simulink model "HvCoorn"  (R2022b)
settings: configuration reference "Icar05FusaMdlCfg" (kept outside this file)
undefined symbols (not defined in the file): BMSActSt_ACChrg, BMSActSt_DCChrg, BMSActSt_disconnect, BMSActSt_offline, BMSActSt_online, BMSActSt_undefined, BMSMainNegRlySt_Clsd_SC, BMSMainNegRlySt_Open_SC, BMSMainNegRlySt_StuckInClsd_SC, BMSMainNegRlySt_StuckInOpen_SC, BMSMainPosRlySt_Clsd_SC, BMSMainPosRlySt_Open_SC, BMSMainPosRlySt_StuckInClsd_SC, BMSPrecRlySt_StuckInOpen_SC, BMSReqSt_ACChrg, BMSReqSt_DCChrg, BMSReqSt_emergencyOffline, BMSReqSt_offline, BMSReqSt_online, Chrg_stCycleBookMod_SC, Chrg_stSingleBookMod_SC, CmpgMod_stInactv_SC, DCDCActSt_buck, DCDCActSt_connected, DCDCActSt_disconnected, DCDCReqSt_buck, DCDCReqSt_standby, EngStrtStop_RefuModDft_SC, EPBActSt_Appld_SC, GearLvr_stDrvGearD_SC, GearLvr_stDrvGearN_SC, GearLvr_stDrvGearP_SC, GearLvr_stDrvGearR_SC, hpp_bACChargeLinkIni_C, hpp_bACChargeLinkOKIni_C, hpp_bAcChgEnaIni_C, hpp_bAcChgPauseIni_C, hpp_bAcLinkTempErrIni_C, hpp_bBattWarmReqIni_C, hpp_bHvilHwErrIni_C, hpp_bHvilStOkIni_C, hpp_bHvRelayClsActIni_C, hpp_bHvRelayOpnActIni_C, hpp_bHvRelayStuckIni_C, hpp_bParked4ChDchgIni_C, hpp_bRemLvBatMntnReqIni_C, hpp_bStartUpReqIni_C, hpp_stHvilCanIni_C, hpp_stWarmTimeCfgRespIni_C, HvCoorn_bAuthEnaSwt_C, HvCoorn_bAuthFailSpdLimOvrd_C, HvCoorn_bAuthFailSpdLimOvrdVal_C, HvCoorn_bAuthStrt_C, HvCoorn_bBMSUnexpdDcnctFailEna_C, HvCoorn_bBuck2RdyBypDCDCEna_C, HvCoorn_bDCChrgFctCfg_C, HvCoorn_bDcChrgWkupEnaChrgLink_C, HvCoorn_bDCDcnct4ACEna_C, HvCoorn_bDCNotBuck2ShtdwnEna_C, HvCoorn_bDrvrLevNotRdyEna_C ... (+295)
libraries: ITKLib x213, simulink x61
(part 6 of 12)

== system HvCoorn/HvCoorn/HVP_HighVoltagePowerOnOffProcedure/A10_ShutDisCh2ShutECUCal ==
  note: Documentation
  HvCoorn_tiHVPStTimer : Inport
  HvCoorn_bHvRlyOpenAct : Inport  Port=2
  icfm_uAct : Inport  Port=3
  icdc_uHvAct : Inport  Port=4
  icfm_stMode : Inport  Port=5
  icrm_stMode : Inport  Port=6
  HvCoorn_bStartUpReq : Inport  Port=7
  HvCoorn_bHvOnFail : Inport  Port=8
  icobc_uHvDcAct : Inport  Port=9
  icfm_bUActSigErr : Inport  Port=10
  icobc_bUHvDcActSigErr : Inport  Port=11
  icdc_bUHvActSigErr : Inport  Port=12
  icbms_uHVBat : Inport  Port=13
  HvCoorn_bHvRlyStuck : Inport  Port=14
  icrm_uAct : Inport  Port=15
  icrm_bUActSigErr : Inport  Port=16
  VehCfg_bFrntMotByp : Inport  Port=17
  icfm_stActvDchrg : Inport  Port=18
  icrm_stActvDchrg : Inport  Port=19
  icisg_uAct : Inport  Port=20
  Add : Sum  Inputs=+-  SaturateOnIntegerOverflow=on
  Copyright : simulink/Model-Wide Utilities/Model Info  Frame=on  DisplayStringWithTags=|  HorizontalTextAlignment=Left  LeftAlignmentValue=0.02
      | © ITK Engineering Technology (Wu Xi) Co., Ltd. (ITKC)
      | 
      | Model Version: %<ModelVersion>
      | Date: %<LastModificationDate>
  FALSE : Constant  Description=FALSE  Value=0  OutDataTypeStr=boolean
      settings: AttributesFormatString=%<Description>
  InlineDescription : ITKLib/Special/InlineDescription  Tag=HideFromReport  Description=主动放电跳转至关ECU  ShowInLibBrowser=0  RefreshPar=0
      settings: SourceProductName=ITKC_Lib
  Logical Operator{1..2,5,11..12} (5 alike) : Logic  AllPortsSameDT=off  OutDataTypeStr=boolean
  Logical Operator3 : Logic  Operator=OR  Inputs=4  AllPortsSameDT=off  OutDataTypeStr=boolean
  Logical Operator4 : Logic  Inputs=3  AllPortsSameDT=off  OutDataTypeStr=boolean
  Logical Operator6 : Logic  Operator=OR  Inputs=4  AllPortsSameDT=off  OutDataTypeStr=boolean
  Logical Operator7 : Logic  Operator=NOT  Inputs=1  AllPortsSameDT=off  OutDataTypeStr=boolean
  Logical Operator8 : Logic  Operator=OR  Inputs=4  AllPortsSameDT=off  OutDataTypeStr=boolean
  Logical Operator9 : Logic  Operator=NOT  Inputs=1  AllPortsSameDT=off  OutDataTypeStr=boolean
  MinMax : MinMax  Function=max  Inputs=5  SaturateOnIntegerOverflow=on
  OR : Logic  Operator=OR  OutDataTypeStr=boolean
  Relational Operator1 : RelationalOperator  OutDataTypeStr=boolean  InputSameDT=off
  Relational Operator{2..3,6,8..10} (6 alike) : RelationalOperator  Operator===  OutDataTypeStr=boolean  InputSameDT=off
  Relational Operator4 : RelationalOperator  OutDataTypeStr=boolean  InputSameDT=off
  Relational Operator5 : RelationalOperator  Operator=>  OutDataTypeStr=boolean  InputSameDT=off
  Relational Operator7 : RelationalOperator  Operator=<  OutDataTypeStr=boolean  InputSameDT=off
  Switch : Switch  Criteria=u2 ~= 0  SaturateOnIntegerOverflow=off  InputSameDT=off
      settings: AttributesFormatString=Criteria : %<Criteria>
  Switch1 : Switch  Criteria=u2 ~= 0  SaturateOnIntegerOverflow=off  InputSameDT=off
      settings: AttributesFormatString=Criteria : %<Criteria>
  Switch2 : Switch  Criteria=u2 ~= 0  SaturateOnIntegerOverflow=off  InputSameDT=off
      settings: AttributesFormatString=Criteria : %<Criteria>
  TRUE : Constant  Description=TRUE  OutDataTypeStr=boolean
      settings: AttributesFormatString=%<Description>
  TRUE1 : Constant  Description=TRUE  OutDataTypeStr=boolean
      settings: AttributesFormatString=%<Description>
  Unit detailed design : simulink/Model-Wide Utilities/DocBlock  Tag=HideFromReport  DocumentType=Text
      content=|
      | SMiVCU-3304 - 电压差大使能高压标志位
      | <电池电压>大于<前电机电压>、<DCDC电压>、<OBC电压>、<后电机电压>超过一定值（HvCoorn_uHvDiffOnThrd_C），则激活[电压差大使能高压标志位]
      |
      | SMiVCU-3303 - MCU主动放电完成标志位
      | <前电机主动放电状态反馈>均为0x1：finished，则激活[MCU主动放电完成标志位]。
      |
      | SMiVCU-3308 - 主动放电跳转至关断ECU标志位
      | [高压继电器断开标志位]为1，且以下任一条件满足，则激活[主动放电跳转至关断ECU标志位]：
      | 1.[MCU主动放电完成标志位]为1；
      | 2.<前电机电压>、<DCDC电压>、<OBC电压>、<后电机电压>均小于一定值（HvCoorn_uMax4Shutdown_C，初始值60V）；
      | 3.<状态持续时间>大于一定值（HvCoorn_tiWait4DchaCanLost_C，5s）；
      | 4.[电压差大使能高压标志位]为1，且[上高压失败标志位]为0，且[上高压需求标志位]为1。
      |
      | SMiVCU-3310 - MCU主动放电失败标志位
      | <前电机主动放电状态反馈>均为0x3：Failure（两驱时屏蔽前电机）则激活[MCU主动放电失败标志位]；
      |
      | SMiVCU-3305 - 主动放电跳转至下电Error标志位
      | 以下任一条件满足，则激活[主动放电跳转至下电Error标志位]：
      | 1.<状态持续时间>大于等于一定值（HvCoorn_tiWait4HvDcha_C，初始值120s）；
      | 2.[高压继电器粘连标志位]为1；
      | 3.[MCU主动放电失败标志位]为1；
  icm_failure : Constant  Description=[8]  Value=MCUActSt_failure  OutDataTypeStr=uint8
      settings: AttributesFormatString=[8]
  icm_failure1 : Constant  Description=[8]  Value=MCUActSt_failure  OutDataTypeStr=uint8
      settings: AttributesFormatString=[8]
  icm_failure2 : Constant  Description=[3]  Value=MCUActvDcgrgSt_Failr_SC  OutDataTypeStr=uint8
      settings: AttributesFormatString=%<Description>
  icm_failure3 : Constant  Description=[3]  Value=MCUActvDcgrgSt_Failr_SC  OutDataTypeStr=uint8
      settings: AttributesFormatString=%<Description>
  icm_failure4 : Constant  Description=[1]  Value=MCUActvDcgrgSt_Cmpl_SC  OutDataTypeStr=uint8
      settings: AttributesFormatString=%<Description>
  icm_failure5 : Constant  Description=[1]  Value=MCUActvDcgrgSt_Cmpl_SC  OutDataTypeStr=uint8
      settings: AttributesFormatString=%<Description>
  sup_bEnaDCUStMan_C : Constant  Description=[0]  Value=HvCoorn_bEnaMCUStMan_C  OutDataTypeStr=boolean
      settings: AttributesFormatString=%<Description>
  sup_tiWait4DchaCanLost_C : Constant  Description=[5]  Value=HvCoorn_tiWait4DchaCanLost_C
      settings: AttributesFormatString=%<Description>
  sup_tiWait4HvDcha_C : Constant  Description=[120]  Value=HvCoorn_tiWait4HvDcha_C
      settings: AttributesFormatString=%<Description>
  sup_uHvDiffOnThres_C : Constant  Description=[70]  Value=HvCoorn_uHvDiffOnThrd_C
      settings: AttributesFormatString=%<Description>
  sup_uIpuShutdown_C : Constant  Description=[60]  Value=HvCoorn_uMax4Shutdown_C
      settings: AttributesFormatString=%<Description>
  HvCoorn_bShutDisCh2ShutECU : Outport  VectorParamsAs1DForOutWhenUnconnected=off
  HvCoorn_bShutDisCh2ShutErr : Outport  Port=2  VectorParamsAs1DForOutWhenUnconnected=off
  bVolDiffEnaHv : Outport  Port=3  VectorParamsAs1DForOutWhenUnconnected=off
  HvCoorn_bMCUActvDchrgCmpl : Outport  Port=4  VectorParamsAs1DForOutWhenUnconnected=off
  HvCoorn_bMCUActvDchrgErr : Outport  Port=5  VectorParamsAs1DForOutWhenUnconnected=off
  wires:
  Logical Operator3/1 -> HvCoorn_bShutDisCh2ShutErr/1  "HvCoorn_bShutDisCh2ShutErr"
  HvCoorn_tiHVPStTimer/1 -> [HvCoorn_tiHVPTimer], Relational Operator4/1
  sup_tiWait4HvDcha_C/1 -> Relational Operator4/2
  HvCoorn_bHvRlyOpenAct/1 -> Logical Operator2/1
  Logical Operator2/1 -> HvCoorn_bShutDisCh2ShutECU/1  "HvCoorn_bShutDisCh2ShutECU"
  sup_uIpuShutdown_C/1 -> Relational Operator7/2
  Relational Operator4/1 -> Logical Operator3/1
  HvCoorn_bHvRlyStuck/1 -> Logical Operator3/2
  icfm_stMode/1 -> Relational Operator2/1
  icm_failure/1 -> Relational Operator2/2
  Logical Operator1/1 -> Logical Operator3/3
  HvCoorn_bStartUpReq/1 -> Logical Operator4/3
  icfm_uAct/1 -> MinMax/1
  icdc_uHvAct/1 -> MinMax/2
  Relational Operator5/1 -> bVolDiffEnaHv/1, Logical Operator4/1
  Relational Operator7/1 -> Logical Operator5/1
  Logical Operator4/1 -> Logical Operator6/4
  Logical Operator6/1 -> Logical Operator2/2
  sup_bEnaDCUStMan_C/1 -> Logical Operator1/2
  HvCoorn_bHvOnFail/1 -> Logical Operator7/1
  Logical Operator7/1 -> Logical Operator4/2
  icobc_uHvDcAct/1 -> MinMax/3
  icbms_uHVBat/1 -> Add/1
  sup_uHvDiffOnThres_C/1 -> Relational Operator5/2
  Add/1 -> Relational Operator5/1
  MinMax/1 -> [HvCoorn_uMaxMCUDCOBC], Relational Operator7/1
  Logical Operator8/1 -> Logical Operator9/1
  icfm_bUActSigErr/1 -> Logical Operator8/1
  icobc_bUHvDcActSigErr/1 -> Logical Operator8/3
  icdc_bUHvActSigErr/1 -> Logical Operator8/2
  Logical Operator9/1 -> Logical Operator5/2
  Relational Operator1/1 -> Logical Operator6/3
  sup_tiWait4DchaCanLost_C/1 -> Relational Operator1/2
  Relational Operator2/1 -> Switch/3
  [HvCoorn_tiHVPTimer] -> Relational Operator1/1
  [HvCoorn_uMaxMCUDCOBC] -> Add/2
  icrm_uAct/1 -> MinMax/4
  icrm_bUActSigErr/1 -> Logical Operator8/4
  icm_failure1/1 -> Relational Operator3/2
  icrm_stMode/1 -> Relational Operator3/1
  Relational Operator3/1 -> OR/2
  OR/1 -> Logical Operator1/1
  Switch/1 -> OR/1
  VehCfg_bFrntMotByp/1 -> [VehCfg_bFrntMotByp], Switch/2
  FALSE/1 -> Switch/1
  TRUE1/1 -> Switch1/1
  icfm_stActvDchrg/1 -> [icfm_stActvDchrg], Relational Operator6/1
  Relational Operator6/1 -> Switch1/3
  icm_failure2/1 -> Relational Operator6/2
  Switch1/1 -> Logical Operator11/1
  icm_failure3/1 -> Relational Operator8/2
  icrm_stActvDchrg/1 -> [icrm_stActvDchrg], Relational Operator8/1
  Relational Operator8/1 -> Logical Operator11/2
  [VehCfg_bFrntMotByp] -> Switch1/2
  [VehCfg_bFrntMotByp] -> Switch2/2
  Relational Operator9/1 -> Switch2/3
  icm_failure4/1 -> Relational Operator9/2
  TRUE/1 -> Switch2/1
  [icfm_stActvDchrg] -> Relational Operator9/1
  Switch2/1 -> Logical Operator12/1
  icm_failure5/1 -> Relational Operator10/2
  [icrm_stActvDchrg] -> Relational Operator10/1
  Relational Operator10/1 -> Logical Operator12/2
  Logical Operator12/1 -> HvCoorn_bMCUActvDchrgCmpl/1, Logical Operator6/1
  Logical Operator11/1 -> Logical Operator3/4, HvCoorn_bMCUActvDchrgErr/1
  Logical Operator5/1 -> Logical Operator6/2
  icisg_uAct/1 -> MinMax/5

== system HvCoorn/HvCoorn/HVP_HighVoltagePowerOnOffProcedure/A11_ShutECU2AftRunCal ==
  note: Documentation
  HvCoorn_tiHVPStTimer : Inport
  icfm_uAct : Inport  Port=2
  HvCoorn_bStartUpReq : Inport  Port=3
  icdc_uHvAct : Inport  Port=4
  icrm_uAct : Inport  Port=5
  Copyright : simulink/Model-Wide Utilities/Model Info  Frame=on  DisplayStringWithTags=|  HorizontalTextAlignment=Left  LeftAlignmentValue=0.02
      | © ITK Engineering Technology (Wu Xi) Co., Ltd. (ITKC)
      | 
      | Model Version: %<ModelVersion>
      | Date: %<LastModificationDate>
  InlineDescription : ITKLib/Special/InlineDescription  Tag=HideFromReport  Description=关断ECU跳转至后运行  ShowInLibBrowser=0  RefreshPar=0
      settings: SourceProductName=ITKC_Lib
  Logical Operator1 : Logic  Inputs=3  AllPortsSameDT=off  OutDataTypeStr=boolean
  Logical Operator2 : Logic  Operator=OR  AllPortsSameDT=off  OutDataTypeStr=boolean
  Logical Operator3 : Logic  Operator=NOT  Inputs=1  AllPortsSameDT=off  OutDataTypeStr=boolean
  Max : MinMax  Function=max  Inputs=2  InputSameDT=on  SaturateOnIntegerOverflow=on
  Relational Operator1 : RelationalOperator  Operator=<  OutDataTypeStr=boolean  InputSameDT=off
  Relational Operator4 : RelationalOperator  OutDataTypeStr=boolean  InputSameDT=off
  Relational Operator7 : RelationalOperator  Operator=<  OutDataTypeStr=boolean  InputSameDT=off
  Unit detailed design : simulink/Model-Wide Utilities/DocBlock  Tag=HideFromReport  DocumentType=Text
      content=|
      | SMiVCU-3306 - 关断ECU跳转至后运行标志位
      | <状态持续时间>大于一定值（HvCoorn_tiShutDownDlyLih_C，初始值20s），或[上高压需求标志位]为0且<前后电机电压>、<DCDC电压>均小于一定值（HvCoorn_uMax4Shutdown_C，初始值60V），则激活[关断ECU跳转至后运行标志位]。
  sup_tiShutDownDlyLih_C : Constant  Description=[20]  Value=HvCoorn_tiShutDownDlyLih_C
      settings: AttributesFormatString=%<Description>
  sup_uIpuShutdown_C : Constant  Description=[60]  Value=HvCoorn_uMax4Shutdown_C
      settings: AttributesFormatString=%<Description>
  HvCoorn_bShutECU2AftRun : Outport  VectorParamsAs1DForOutWhenUnconnected=off
  wires:
  Logical Operator2/1 -> HvCoorn_bShutECU2AftRun/1  "HvCoorn_bShutECU2AftRun"
  icfm_uAct/1 -> Max/1
  sup_uIpuShutdown_C/1 -> Relational Operator7/2, Relational Operator1/2
  sup_tiShutDownDlyLih_C/1 -> Relational Operator4/2
  HvCoorn_tiHVPStTimer/1 -> Relational Operator4/1
  Relational Operator7/1 -> Logical Operator1/2
  Relational Operator4/1 -> Logical Operator2/2
  HvCoorn_bStartUpReq/1 -> Logical Operator3/1
  Logical Operator3/1 -> Logical Operator1/1
  Logical Operator1/1 -> Logical Operator2/1
  icdc_uHvAct/1 -> Relational Operator1/1
  Relational Operator1/1 -> Logical Operator1/3
  icrm_uAct/1 -> Max/2
  Max/1 -> Relational Operator7/1

== system HvCoorn/HvCoorn/HVP_HighVoltagePowerOnOffProcedure/A12_ShutECU2CommCal ==
  note: Documentation
  bVolDiffEnaHv : Inport
  HvCoorn_bStartUpReq : Inport  Port=2
  HvCoorn_bHvOnFail : Inport  Port=3
  HvCoorn_bDischargeErrOld : Inport  Port=4
  HvCoorn_bHvInitFail : Inport  Port=5
  Copyright : simulink/Model-Wide Utilities/Model Info  Frame=on  DisplayStringWithTags=|  HorizontalTextAlignment=Left  LeftAlignmentValue=0.02
      | © ITK Engineering Technology (Wu Xi) Co., Ltd. (ITKC)
      | 
      | Model Version: %<ModelVersion>
      | Date: %<LastModificationDate>
  InlineDescription : ITKLib/Special/InlineDescription  Tag=HideFromReport  Description=关断ECU跳转至通讯准备  ShowInLibBrowser=0  RefreshPar=0
      settings: SourceProductName=ITKC_Lib
  Logical Operator1 : Logic  Inputs=5  AllPortsSameDT=off  OutDataTypeStr=boolean
  Logical Operator2 : Logic  Operator=NOT  Inputs=1  AllPortsSameDT=off  OutDataTypeStr=boolean
  Logical Operator3 : Logic  Operator=NOT  Inputs=1  AllPortsSameDT=off  OutDataTypeStr=boolean
  Logical Operator4 : Logic  Operator=NOT  Inputs=1  AllPortsSameDT=off  OutDataTypeStr=boolean
  Unit detailed design : simulink/Model-Wide Utilities/DocBlock  Tag=HideFromReport  DocumentType=Text
      content=|
      | SMiVCU-3309 - 关断ECU跳转至通讯准备标志位
      | 以下条件全部满足，则激活[关断ECU跳转至通讯准备标志位]：
      | 1.[上高压需求标志位]为1；
      | 2.[上高压失败标志位]为0；
      | 3.[MCU主动放电失败标志位]为0；
      | 4.[高压初始化失败标志位]为0；
      | 5.[电压差大使能高压标志位]为1；
  HvCoorn_bShutECU2Comm : Outport  VectorParamsAs1DForOutWhenUnconnected=off
  wires:
  HvCoorn_bHvOnFail/1 -> Logical Operator3/1
  HvCoorn_bDischargeErrOld/1 -> Logical Operator4/1
  HvCoorn_bStartUpReq/1 -> Logical Operator1/1
  Logical Operator3/1 -> Logical Operator1/2
  Logical Operator4/1 -> Logical Operator1/3
  Logical Operator1/1 -> HvCoorn_bShutECU2Comm/1  "HvCoorn_bShutECU2Comm"
  HvCoorn_bHvInitFail/1 -> Logical Operator2/1
  Logical Operator2/1 -> Logical Operator1/4
  bVolDiffEnaHv/1 -> Logical Operator1/5

== system HvCoorn/HvCoorn/HVP_HighVoltagePowerOnOffProcedure/A13_AftRun2NetManCal ==
  note: Documentation
  HvCoorn_tiHVPTimer : Inport
  HvCoorn_bStartUpReq : Inport  Port=2
  EngStrtStop_stRefuMod : Inport  Port=3
  Calibration1 : Constant  Description=[0]  Value=EngStrtStop_RefuModDft_SC  SampleTime=-1
      settings: AttributesFormatString=%<Description>
  Calibration2 : Constant  Description=[300]  Value=HvCoorn_tiRefuModOvti2NetManDly_C  SampleTime=-1
      settings: AttributesFormatString=%<Description>
  Copyright : simulink/Model-Wide Utilities/Model Info  Frame=on  DisplayStringWithTags=|  HorizontalTextAlignment=Left  LeftAlignmentValue=0.02
      | © ITK Engineering Technology (Wu Xi) Co., Ltd. (ITKC)
      | 
      | Model Version: %<ModelVersion>
      | Date: %<LastModificationDate>
  Equal1 : RelationalOperator  Operator===  OutDataTypeStr=boolean
  InlineDescription : ITKLib/Special/InlineDescription  Tag=HideFromReport  Description=后运行跳转至网络保持  ShowInLibBrowser=0  RefreshPar=0
      settings: SourceProductName=ITKC_Lib
  Logical Operator5 : Logic  Operator=NOT  Inputs=1  AllPortsSameDT=off  OutDataTypeStr=boolean
  Logical Operator6 : Logic  Inputs=3  AllPortsSameDT=off  OutDataTypeStr=boolean
  Not : Logic  Operator=NOT  AllPortsSameDT=off  OutDataTypeStr=boolean
  OR : Logic  Operator=OR  Inputs=3  OutDataTypeStr=boolean
  Relational Operator4 : RelationalOperator  Operator=>  OutDataTypeStr=boolean  InputSameDT=off
  TaskTime_s3 : Constant  Value=TaskTime_10ms
      settings: AttributesFormatString=[0.01]
  TurnOnDelayVari1 : ITKLib/TimeCounter/TurnOnDelayVari
      settings: AttributesFormatString=TurnOnDelay  SourceProductName=ITKC_Lib
  Unit detailed design : simulink/Model-Wide Utilities/DocBlock  Tag=HideFromReport  DocumentType=Text
      content=|
      | SMiVCU-3313 - 后运行跳转至网络保持标志位
      | <状态持续时间>大于一定值（HvCoorn_tiWaitChrgFullShutdown_C，1s）且[上高压需求标志位]为0，则激活[后运行跳转至网络保持标志位]。
  sup_tiWaitChgFullShutdown_C : Constant  Description=[1]  Value=HvCoorn_tiWaitChrgFullShutdown_C
      settings: AttributesFormatString=%<Description>
  sup_tiWaitChgFullShutdown_C1 : Constant  Description=[0]  Value=HvCoorn_bRefuModOvti2NetManShd_C
      settings: AttributesFormatString=%<Description>
  HvCoorn_bAftRun2NetMan : Outport  VectorParamsAs1DForOutWhenUnconnected=off
  wires:
  HvCoorn_tiHVPTimer/1 -> Relational Operator4/1
  sup_tiWaitChgFullShutdown_C/1 -> Relational Operator4/2
  Relational Operator4/1 -> Logical Operator6/1
  HvCoorn_bStartUpReq/1 -> Logical Operator5/1
  Logical Operator6/1 -> HvCoorn_bAftRun2NetMan/1  "HvCoorn_bAftRun2NetMan"
  Logical Operator5/1 -> Logical Operator6/2
  EngStrtStop_stRefuMod/1 -> Equal1/1
  Calibration1/1 -> Equal1/2
  Equal1/1 -> OR/2, Not/1
  Calibration2/1 -> TurnOnDelayVari1/3
  TaskTime_s3/1 -> TurnOnDelayVari1/2
  Not/1 -> TurnOnDelayVari1/1
  TurnOnDelayVari1/1 -> OR/3
  OR/1 -> Logical Operator6/3
  sup_tiWaitChgFullShutdown_C1/1 -> OR/1

== system HvCoorn/HvCoorn/HVP_HighVoltagePowerOnOffProcedure/A14_NetMan2PwrShutCal ==
  VCCM_bNetMaintn : Inport
  HvCoorn_tiHVPStTimer : Inport  Port=2
  HvCoorn_stHVPOld : Inport  Port=3
  AND : Logic  OutDataTypeStr=boolean
  Logical Operator4 : Logic  Operator=OR  Inputs=3  AllPortsSameDT=off  OutDataTypeStr=boolean
  Not : Logic  Operator=NOT  AllPortsSameDT=off  OutDataTypeStr=boolean
  Relational Operator15 : RelationalOperator  Operator===  OutDataTypeStr=boolean  InputSameDT=off
  Relational Operator4 : RelationalOperator  Operator=>  OutDataTypeStr=boolean  InputSameDT=off
  Wait4MindChange : Constant  Value=125  OutDataTypeStr=uint8
  sup_bLlswShutDownMan_C : Constant  Description=[0]  Value=HvCoorn_bLlswShutDownMan_C  OutDataTypeStr=boolean
      settings: AttributesFormatString=%<Description>
  sup_tiTimeOutStandbyRdyHv_C : Constant  Description=[120]  Value=HvCoorn_tiTimeOutNetMan_C
      settings: AttributesFormatString=%<Description>
  HvCoorn_bNetMan2PwrShut : Outport  VectorParamsAs1DForOutWhenUnconnected=off
  wires:
  VCCM_bNetMaintn/1 -> Not/1
  sup_bLlswShutDownMan_C/1 -> Logical Operator4/2
  Logical Operator4/1 -> HvCoorn_bNetMan2PwrShut/1  "HvCoorn_bNetMan2PwrShut"
  Not/1 -> Logical Operator4/1
  HvCoorn_tiHVPStTimer/1 -> Relational Operator4/1
  Relational Operator4/1 -> AND/1
  Relational Operator15/1 -> AND/2
  AND/1 -> Logical Operator4/3
  HvCoorn_stHVPOld/1 -> Relational Operator15/1
  sup_tiTimeOutStandbyRdyHv_C/1 -> Relational Operator4/2
  Wait4MindChange/1 -> Relational Operator15/2

== system HvCoorn/HvCoorn/HVP_HighVoltagePowerOnOffProcedure/A15_Wake2NetManCal ==
  note: Documentation
  HvCoorn_bStartUpReq : Inport
  HvCoorn_tiHVPTimer : Inport  Port=2
  Copyright : simulink/Model-Wide Utilities/Model Info  Frame=on  DisplayStringWithTags=|  HorizontalTextAlignment=Left  LeftAlignmentValue=0.02
      | © ITK Engineering Technology (Wu Xi) Co., Ltd. (ITKC)
      | 
      | Model Version: %<ModelVersion>
      | Date: %<LastModificationDate>
  InlineDescription : ITKLib/Special/InlineDescription  Tag=HideFromReport  Description=唤醒跳转至网络保持  ShowInLibBrowser=0  RefreshPar=0
      settings: SourceProductName=ITKC_Lib
  Logical Operator2 : Logic  AllPortsSameDT=off  OutDataTypeStr=boolean
  Logical Operator5 : Logic  Operator=NOT  Inputs=1  AllPortsSameDT=off  OutDataTypeStr=boolean
  Relational Operator4 : RelationalOperator  Operator=>  OutDataTypeStr=boolean  InputSameDT=off
  Unit detailed design : simulink/Model-Wide Utilities/DocBlock  Tag=HideFromReport  DocumentType=Text
      content=|
      | <状态持续时间>大于一定值（HvCoorn_tiKeyOnChk_C，0.05s）且[上高压需求标志位]为0，则激活[唤醒至网络保持标志位]。
  sup_tiKeyOnCheck_C : Constant  Description=[5]  Value=HvCoorn_tiKeyOnChk_C
      settings: AttributesFormatString=%<Description>
  HvCoorn_bWake2NetMan : Outport  VectorParamsAs1DForOutWhenUnconnected=off
  wires:
  HvCoorn_bStartUpReq/1 -> Logical Operator5/1
  Logical Operator2/1 -> HvCoorn_bWake2NetMan/1  "HvCoorn_bWake2NetMan"
  HvCoorn_tiHVPTimer/1 -> Relational Operator4/1
  sup_tiKeyOnCheck_C/1 -> Relational Operator4/2
  Logical Operator5/1 -> Logical Operator2/1
  Relational Operator4/1 -> Logical Operator2/2

== system HvCoorn/HvCoorn/HVP_HighVoltagePowerOnOffProcedure/A16_Init2AftRunCal ==
  note: Documentation
  HvCoorn_bStartUpReq : Inport
  HvCoorn_tiHVPTimer : Inport  Port=2
  Copyright : simulink/Model-Wide Utilities/Model Info  Frame=on  DisplayStringWithTags=|  HorizontalTextAlignment=Left  LeftAlignmentValue=0.02
      | © ITK Engineering Technology (Wu Xi) Co., Ltd. (ITKC)
      | 
      | Model Version: %<ModelVersion>
      | Date: %<LastModificationDate>
  InlineDescription : ITKLib/Special/InlineDescription  Tag=HideFromReport  Description=初始化跳转至后运行  ShowInLibBrowser=0  RefreshPar=0
      settings: SourceProductName=ITKC_Lib
  Logical Operator2 : Logic  AllPortsSameDT=off  OutDataTypeStr=boolean
  Logical Operator5 : Logic  Operator=NOT  Inputs=1  AllPortsSameDT=off  OutDataTypeStr=boolean
  Relational Operator4 : RelationalOperator  Operator=>  OutDataTypeStr=boolean  InputSameDT=off
  Unit detailed design : simulink/Model-Wide Utilities/DocBlock  Tag=HideFromReport  DocumentType=Text
      content=|
      | <状态持续时间>大于一定值（HvCoorn_tiWaitIgnOff_C，5s）且[上高压需求标志位]为0，则激活[初始化跳转至后运行标志位]。
  sup_tiWaitIgnOff_C : Constant  Description=[5]  Value=HvCoorn_tiWaitIgnOff_C
      settings: AttributesFormatString=%<Description>
  HvCoorn_bInit2AftRun : Outport  VectorParamsAs1DForOutWhenUnconnected=off
  wires:
  Relational Operator4/1 -> Logical Operator2/2
  Logical Operator5/1 -> Logical Operator2/1
  sup_tiWaitIgnOff_C/1 -> Relational Operator4/2
  HvCoorn_tiHVPTimer/1 -> Relational Operator4/1
  Logical Operator2/1 -> HvCoorn_bInit2AftRun/1  "HvCoorn_bInit2AftRun"
  HvCoorn_bStartUpReq/1 -> Logical Operator5/1

== system HvCoorn/HvCoorn/HVP_HighVoltagePowerOnOffProcedure/A17_EmergencyShutDownCal ==
  note: Documentation
  HvCoorn_tiHVPStTimer : Inport
  HvCoorn_bHvRlyStuck : Inport  Port=2
  HvCoorn_bHvRlyOpenAct : Inport  Port=3
  icfm_uAct : Inport  Port=4
  icdc_uHvAct : Inport  Port=5
  icfm_stMode : Inport  Port=6
  icbms_iHVBat : Inport  Port=7
  HvCoorn_bStartUpReq : Inport  Port=8
  icfm_nAct : Inport  Port=9
  HvCoorn_stHVPOld : Inport  Port=10
  ved_bHvShtdwn : Inport  Port=11
  icobc_uHvDcAct : Inport  Port=12
  icfm_bUActSigErr : Inport  Port=13
  icobc_bUHvDcActSigErr : Inport  Port=14
  icdc_bUHvActSigErr : Inport  Port=15
  icrm_nAct : Inport  Port=16
  icrm_bUActSigErr : Inport  Port=17
  icrm_uAct : Inport  Port=18
  icrm_stMode : Inport  Port=19
  HvCoorn_bMCUActvDchrgCmpl : Inport  Port=20
  HvCoorn_bMCUActvDchrgErr : Inport  Port=21
  Abs : Abs
  Abs1 : Abs
  Abs2 : Abs
  Copyright : simulink/Model-Wide Utilities/Model Info  Frame=on  DisplayStringWithTags=|  HorizontalTextAlignment=Left  LeftAlignmentValue=0.02
      | © ITK Engineering Technology (Wu Xi) Co., Ltd. (ITKC)
      | 
      | Model Version: %<ModelVersion>
      | Date: %<LastModificationDate>
  EmWait4KeyOff : Constant  Description=EmWait4KeyOff  Value=156  OutDataTypeStr=uint8
      settings: AttributesFormatString=|
      | %<OutDataTypeStr>
      | %<Description>
  InlineDescription : ITKLib/Special/InlineDescription  Tag=HideFromReport  Description=紧急下电  ShowInLibBrowser=0  RefreshPar=0
      settings: SourceProductName=ITKC_Lib
  Logical Operator1 : Logic  Operator=OR  Inputs=3  AllPortsSameDT=off  OutDataTypeStr=boolean
  Logical Operator{4,6,8,11} (4 alike) : Logic  AllPortsSameDT=off  OutDataTypeStr=boolean
  Logical Operator12 : Logic  Operator=OR  Inputs=4  AllPortsSameDT=off  OutDataTypeStr=boolean
  Logical Operator13 : Logic  Operator=NOT  Inputs=1  AllPortsSameDT=off  OutDataTypeStr=boolean
  Logical Operator2 : Logic  Operator=NOT  Inputs=1  AllPortsSameDT=off  OutDataTypeStr=boolean
  Logical Operator3 : Logic  Operator=OR  Inputs=4  AllPortsSameDT=off  OutDataTypeStr=boolean
  Logical Operator5 : Logic  Operator=OR  AllPortsSameDT=off  OutDataTypeStr=boolean
  Logical Operator7 : Logic  Operator=NOT  Inputs=1  AllPortsSameDT=off  OutDataTypeStr=boolean
  Logical Operator9 : Logic  Inputs=3  AllPortsSameDT=off  OutDataTypeStr=boolean
  Max : MinMax  Function=max  Inputs=2  InputSameDT=on  SaturateOnIntegerOverflow=on
  MinMax : MinMax  Function=max  Inputs=4  SaturateOnIntegerOverflow=on
  OR : Logic  Operator=OR  OutDataTypeStr=boolean
  OR1 : Logic  Operator=OR  OutDataTypeStr=boolean
  Relational Operator1 : RelationalOperator  OutDataTypeStr=boolean  InputSameDT=off
  Relational Operator10 : RelationalOperator  Operator=<=  OutDataTypeStr=boolean  InputSameDT=off
  Relational Operator11 : RelationalOperator  Operator=<  OutDataTypeStr=boolean  InputSameDT=off
  Relational Operator2 : RelationalOperator  OutDataTypeStr=boolean  InputSameDT=off
  Relational Operator3 : RelationalOperator  Operator===  OutDataTypeStr=boolean  InputSameDT=off
  Relational Operator4 : RelationalOperator  Operator=>  OutDataTypeStr=boolean  InputSameDT=off
  Relational Operator5 : RelationalOperator  OutDataTypeStr=boolean  InputSameDT=off
  Relational Operator6 : RelationalOperator  Operator=>  OutDataTypeStr=boolean  InputSameDT=off
  Relational Operator7 : RelationalOperator  Operator=>  OutDataTypeStr=boolean  InputSameDT=off
  Relational Operator8 : RelationalOperator  Operator=<  OutDataTypeStr=boolean  InputSameDT=off
  Relational Operator9 : RelationalOperator  Operator===  OutDataTypeStr=boolean  InputSameDT=off
  Unit detailed design : simulink/Model-Wide Utilities/DocBlock  Tag=HideFromReport  DocumentType=Text
      content=|
      | SMiVCU-3320 - 紧急下电初始化跳转至断高压标志位
      | <电池电流>的绝对值小于一定值（HvCoorn_iBatMax4RlyOpen_C，5s）或<状态持续时间>大于一定值（HvCoorn_tiHvOpenDlyEmerg_C，5s），则激活[紧急下电初始化跳转至断高压标志位]。
      |
      |
      | SMiVCU-3321 - 紧急下电放电跳转至放电Error标志位
      | 以下任一条件满足，则激活[紧急下电放电跳转至放电Error标志位]：
      | 1.<状态持续时间>大于一定值（HvCoorn_tiWait4HvDcha_C，120s）；
      | 2.[MCU主动放电失败标志位]为1；
      | 3.[高压继电器粘连标志位]为1；
      |
      | SMiVCU-3329 - 紧急下电等待KeyOff跳转至网络保持标志位
      | <状态持续时间>大于一定值（HvCoorn_tiWait4LlswEolShutdown_C，10s）且[上高压需求标志位]为0，则激活[紧急下电等待KeyOff跳转至网络保持标志位]。
      |
      | SMiVCU-3327 - 紧急下电放电跳转至等待KeyOff标志位
      | 以下条件全部满足，则激活[紧急下电放电跳转至等待KeyOff标志位]：
      | 1.[MCU主动放电完成标志位]为1；
      | 2.<前电机电压>、<DCDC电压>、<OBC电压>、<后电机电压>均小于一定值（HvCoorn_uThd4EmergShutdown_C，初始值60V）；
      | 3.<状态持续时间>大于一定值（HvCoorn_tiWait4DchaCanLost_C，5s）；
      |
      | SMiVCU-3331 - 紧急下电退出标志位
      | 满足以下全部条件，则激活[紧急下电退出标志位]:
      | 1.[紧急下电放电跳转至等待KeyOff标志位]为1；
      | 2.上一时刻<高压系统状态>大于156；
      | 3.[下电请求标志位]为0；
      |
      | SMiVCU-3333 - 紧急下电断高压跳转至主动放电标志位
      | [高压继电器断开标志位]为1，且<前后电机转速>的绝对值均小于一定值（HvCoorn_nMotThrd4DChrg_C，60rpm），则激活[紧急下电断高压跳转至主动放电标志位]
  icm_failure : Constant  Description=[8]  Value=MCUActSt_failure  OutDataTypeStr=uint8
      settings: AttributesFormatString=[8]
  icm_failure1 : Constant  Description=[8]  Value=MCUActSt_failure  OutDataTypeStr=uint8
      settings: AttributesFormatString=[8]
  sup_bEmEnaDCUStMan_C : Constant  Description=[0]  Value=HvCoorn_bEmEnaMCUStMan_C  OutDataTypeStr=boolean
      settings: AttributesFormatString=%<Description>
  sup_iBatMax4RlyOpn_C : Constant  Description=[5]  Value=HvCoorn_iBatMax4RlyOpen_C
      settings: AttributesFormatString=%<Description>
  sup_nMotThres4Dcha_C : Constant  Description=[30000]  Value=HvCoorn_nMotEmShutHv2DChrg_C
      settings: AttributesFormatString=%<Description>
  sup_tiHvesOpDlyEmerg_C : Constant  Description=[0.2]  Value=HvCoorn_tiHvOpenDlyEmerg_C
      settings: AttributesFormatString=%<Description>
  sup_tiWait4DchaCanLost_C : Constant  Description=[5]  Value=HvCoorn_tiWait4DchaCanLost_C
      settings: AttributesFormatString=%<Description>
  sup_tiWait4HvDcha_C : Constant  Description=[120]  Value=HvCoorn_tiWait4HvDcha_C
      settings: AttributesFormatString=%<Description>
  sup_tiWait4LlswEolShutdown_C : Constant  Description=[10]  Value=HvCoorn_tiWait4LlswEolShutdown_C
      settings: AttributesFormatString=%<Description>
  sup_tiWait4LlswEolShutdown_C1 : Constant  Description=[0.2]  Value=HvCoorn_tiWait4EmShutHv2DChrg_C
      settings: AttributesFormatString=%<Description>
  sup_uThresEmerg_C : Constant  Description=[60]  Value=HvCoorn_uThd4EmergShutdown_C
      settings: AttributesFormatString=%<Description>
  HvCoorn_bEmIni2ShutHV : Outport  VectorParamsAs1DForOutWhenUnconnected=off
  HvCoorn_bEmShutHv2DisCh : Outport  Port=2  VectorParamsAs1DForOutWhenUnconnected=off
  HvCoorn_bEmDisCh2WaitKeyOff : Outport  Port=3  VectorParamsAs1DForOutWhenUnconnected=off
  HvCoorn_bEmDisCh2Err : Outport  Port=4  VectorParamsAs1DForOutWhenUnconnected=off
  HvCoorn_bEmWaitKeyOff2NetMan : Outport  Port=5  VectorParamsAs1DForOutWhenUnconnected=off
  HvCoorn_bEmShutHeal : Outport  Port=6  VectorParamsAs1DForOutWhenUnconnected=off
  wires:
  sup_tiHvesOpDlyEmerg_C/1 -> Relational Operator4/2
  Logical Operator5/1 -> HvCoorn_bEmIni2ShutHV/1
  sup_tiWait4HvDcha_C/1 -> Relational Operator2/2
  Logical Operator3/1 -> HvCoorn_bEmDisCh2Err/1
  sup_tiWait4LlswEolShutdown_C/1 -> Relational Operator7/2
  Logical Operator1/1 -> HvCoorn_bEmDisCh2WaitKeyOff/1, Logical Operator9/1
  Relational Operator2/1 -> Logical Operator3/1
  HvCoorn_bHvRlyStuck/1 -> Logical Operator3/3
  icfm_stMode/1 -> Relational Operator9/1
  icm_failure/1 -> Relational Operator9/2
  Logical Operator6/1 -> Logical Operator3/4
  sup_nMotThres4Dcha_C/1 -> Relational Operator10/2
  Abs/1 -> Max/1
  icfm_nAct/1 -> Abs/1
  Relational Operator10/1 -> Logical Operator4/2
  HvCoorn_bHvRlyOpenAct/1 -> Logical Operator4/1
  sup_iBatMax4RlyOpn_C/1 -> Relational Operator11/2
  Abs1/1 -> Relational Operator11/1
  icbms_iHVBat/1 -> Abs1/1
  Relational Operator11/1 -> Logical Operator5/1
  Relational Operator4/1 -> Logical Operator5/2
  sup_bEmEnaDCUStMan_C/1 -> Logical Operator6/2
  Relational Operator9/1 -> OR/1
  HvCoorn_bStartUpReq/1 -> Logical Operator7/1
  Relational Operator7/1 -> Logical Operator8/1
  Logical Operator8/1 -> HvCoorn_bEmWaitKeyOff2NetMan/1
  Logical Operator7/1 -> Logical Operator8/2
  EmWait4KeyOff/1 -> Relational Operator1/2
  HvCoorn_stHVPOld/1 -> Relational Operator1/1
  ved_bHvShtdwn/1 -> Logical Operator2/1
  Relational Operator1/1 -> Logical Operator9/2
  Logical Operator2/1 -> Logical Operator9/3
  Logical Operator9/1 -> HvCoorn_bEmShutHeal/1
  sup_uThresEmerg_C/1 -> Relational Operator8/2
  icfm_uAct/1 -> MinMax/1
  icdc_uHvAct/1 -> MinMax/2
  Relational Operator8/1 -> Logical Operator11/1
  icobc_uHvDcAct/1 -> MinMax/3
  MinMax/1 -> Relational Operator8/1
  Logical Operator12/1 -> Logical Operator13/1
  icfm_bUActSigErr/1 -> Logical Operator12/1
  icobc_bUHvDcActSigErr/1 -> Logical Operator12/3
  icdc_bUHvActSigErr/1 -> Logical Operator12/2
  Logical Operator13/1 -> Logical Operator11/2
  sup_tiWait4DchaCanLost_C/1 -> Relational Operator5/2
  HvCoorn_tiHVPStTimer/1 -> [HvCoorn_tiHVPTimer], Relational Operator2/1, Relational Operator4/1
  [HvCoorn_tiHVPTimer] -> Relational Operator7/1
  [HvCoorn_tiHVPTimer] -> Relational Operator5/1
  icrm_nAct/1 -> Abs2/1
  Abs2/1 -> Max/2
  Max/1 -> Relational Operator10/1
  icrm_bUActSigErr/1 -> Logical Operator12/4
  icrm_uAct/1 -> MinMax/4
  icm_failure1/1 -> Relational Operator3/2
  icrm_stMode/1 -> Relational Operator3/1
  Relational Operator3/1 -> OR/2
  OR/1 -> Logical Operator6/1
  HvCoorn_bMCUActvDchrgErr/1 -> Logical Operator3/2
  HvCoorn_bMCUActvDchrgCmpl/1 -> Logical Operator1/1
  Logical Operator11/1 -> Logical Operator1/2
  Relational Operator5/1 -> Logical Operator1/3
  [HvCoorn_tiHVPTimer] -> Relational Operator6/1
  sup_tiWait4LlswEolShutdown_C1/1 -> Relational Operator6/2
  Logical Operator4/1 -> OR1/1
  Relational Operator6/1 -> OR1/2
  OR1/1 -> HvCoorn_bEmShutHv2DisCh/1

== system HvCoorn/HvCoorn/HVP_HighVoltagePowerOnOffProcedure/A18_ShutDownReqCal ==
  note: This subsystem calculates vehicle high voltage shut down flag and emergency shut down flag, based on vehicle eror level signal.
  note: Documentation
  ved_bEmgcyHvShtdwn : Inport
  HvCoorn_stHVPOld : Inport  Port=2
  Copyright : simulink/Model-Wide Utilities/Model Info  Frame=on  DisplayStringWithTags=|  HorizontalTextAlignment=Left  LeftAlignmentValue=0.02
      | © ITK Engineering Technology (Wu Xi) Co., Ltd. (ITKC)
      | 
      | Model Version: %<ModelVersion>
      | Date: %<LastModificationDate>
  InlineDescription : ITKLib/Special/InlineDescription  Tag=HideFromReport  Description=故障下高压  ShowInLibBrowser=0  RefreshPar=0
      settings: SourceProductName=ITKC_Lib
  Logical Operator1 : Logic  Inputs=3  AllPortsSameDT=off  OutDataTypeStr=boolean
  NormShut2 : Constant  Description=HvContactorRequest  Value=12  OutDataTypeStr=uint8
      settings: AttributesFormatString=|
      | %<OutDataTypeStr>
      | %<Description>
  NormShut3 : Constant  Description=Shutdown_HV  Value=101  OutDataTypeStr=uint8
      settings: AttributesFormatString=|
      | %<OutDataTypeStr>
      | %<Description>
  Relational Operator12 : RelationalOperator  OutDataTypeStr=boolean  InputSameDT=off
  Relational Operator3 : RelationalOperator  Operator=<=  OutDataTypeStr=boolean  InputSameDT=off
  Unit detailed design : simulink/Model-Wide Utilities/DocBlock  Tag=HideFromReport  DocumentType=Text
      content=|
      | SMiVCU-3772 - 故障下高压
      | 若<整车故障等级>大于等于4，则激活[下电请求标志位]。
      |
      | 若<整车故障等级>等于5，且上一时刻<高压系统状态>在12~101之间，则激活[紧急下电请求]
  HvCoorn_bEmgcyShutDownReq : Outport  VectorParamsAs1DForOutWhenUnconnected=off
  wires:
  Logical Operator1/1 -> HvCoorn_bEmgcyShutDownReq/1
  NormShut2/1 -> Relational Operator12/2
  HvCoorn_stHVPOld/1 -> Relational Operator12/1, Relational Operator3/1
  Relational Operator12/1 -> Logical Operator1/2
  NormShut3/1 -> Relational Operator3/2
  Relational Operator3/1 -> Logical Operator1/3
  ved_bEmgcyHvShtdwn/1 -> Logical Operator1/1

== system HvCoorn/HvCoorn/HVP_HighVoltagePowerOnOffProcedure/A20_HVPStOvrd ==
  HvCoorn_stHVPRaw : Inport
  Switch : Switch  Criteria=u2 ~= 0  SaturateOnIntegerOverflow=off  InputSameDT=off
      settings: AttributesFormatString=Criteria : %<Criteria>
  ocm_standby1 : Constant  Description=[90]  Value=HvCoorn_noHVStOvrdVal_C  OutDataTypeStr=uint8
      settings: AttributesFormatString=%<Description>
  ocm_standby2 : Constant  Description=[0]  Value=HvCoorn_bHVStOvrd_C
      settings: AttributesFormatString=%<Description>
  HvCoorn_stHVP : Outport
  wires:
  HvCoorn_stHVPRaw/1 -> Switch/3
  Switch/1 -> HvCoorn_stHVP/1
  ocm_standby2/1 -> Switch/2
  ocm_standby1/1 -> Switch/1

== system HvCoorn/HvCoorn/HVP_HighVoltagePowerOnOffProcedure/A21_ShutDwnEna ==
  HvCoorn_stHVP : Inport
  Equal{,1..3} (4 alike) : RelationalOperator  Operator===  OutDataTypeStr=boolean  RndMeth=Simplest  InputSameDT=off
  OR : Logic  Operator=OR  Inputs=3  OutDataTypeStr=boolean
  OR1 : Logic  Operator=OR  OutDataTypeStr=boolean
  uint1 : Constant  Description=""  Value=125  OutDataTypeStr=uint8
      settings: AttributesFormatString=|
      | %<OutDataTypeStr>
      | %<Description>
  uint2 : Constant  Description=""  Value=130  OutDataTypeStr=uint8
      settings: AttributesFormatString=|
      | %<OutDataTypeStr>
      | %<Description>
  uint3 : Constant  Description=""  Value=158  OutDataTypeStr=uint8
      settings: AttributesFormatString=|
      | %<OutDataTypeStr>
      | %<Description>
  uint4 : Constant  Description=""  Value=160  OutDataTypeStr=uint8
      settings: AttributesFormatString=|
      | %<OutDataTypeStr>
      | %<Description>
  HvCoorn_bAllwShutNet : Outport
  HvCoorn_bAllwSlep : Outport  Port=2
  wires:
  HvCoorn_stHVP/1 -> Equal1/1, Equal3/1, Equal2/1, Equal/1
  uint1/1 -> Equal/2
  uint2/1 -> Equal1/2
  uint3/1 -> Equal2/2
  uint4/1 -> Equal3/2
  Equal/1 -> OR/1
  Equal1/1 -> OR1/2
  Equal2/1 -> OR/2
  Equal3/1 -> OR1/1
  OR/1 -> HvCoorn_bAllwShutNet/1
  OR1/1 -> OR/3, HvCoorn_bAllwSlep/1

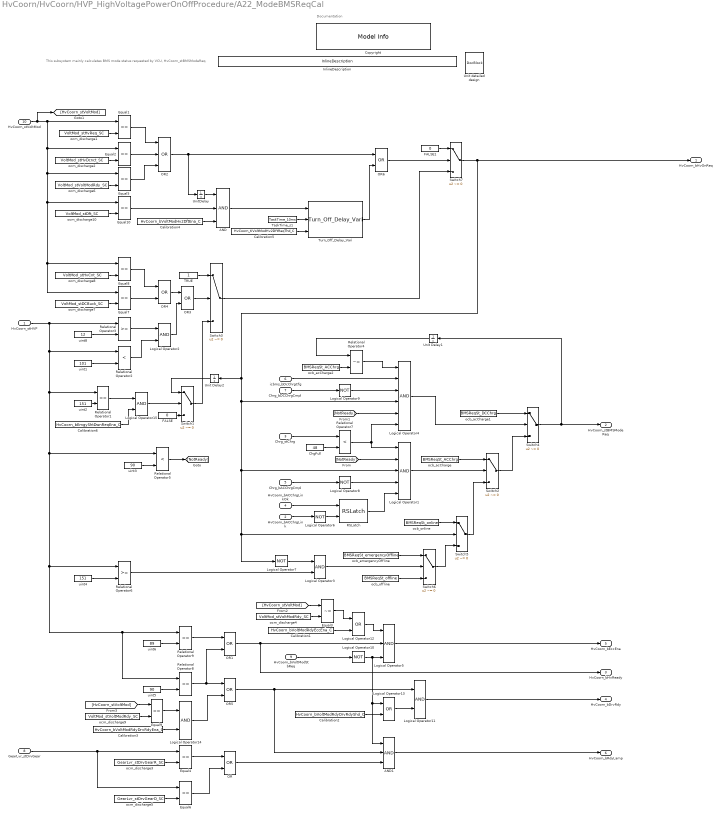
== system HvCoorn/HvCoorn/HVP_HighVoltagePowerOnOffProcedure/A22_ModeBMSReqCal ==
  note: This subsystem mainly calculates BMS mode status requested by VCU, HvCoorn_stBMSModeReq.
  note: Documentation
  HvCoorn_stHVP : Inport
  HvCoorn_bACChrgLink : Inport  Port=2
  Chrg_stChrg : Inport  Port=3
  HvCoorn_bACChrgLinkOk : Inport  Port=4
  Chrg_bACChrgCmpl : Inport  Port=5
  icbms_bDcChrgCfg : Inport  Port=6
  Chrg_bDCChrgCmpl : Inport  Port=7
  GearLvr_stDrvGear : Inport  Port=8
  HvCoorn_bVoltModStbReq : Inport  Port=9
  HvCoorn_stVoltMod : Inport  Port=10
  AND : Logic  Inputs=3  OutDataTypeStr=boolean
  AND1 : Logic  Inputs=3  OutDataTypeStr=boolean
  Calibration1 : Constant  Description=[1]  Value=HvCoorn_bVoltModRdyEccEna_C  SampleTime=-1
      settings: AttributesFormatString=%<Description>
  Calibration2 : Constant  Description=[0]  Value=HvCoorn_bVoltModRdyDrvRdyShd_C  SampleTime=-1
      settings: AttributesFormatString=%<Description>
  Calibration3 : Constant  Description=[0]  Value=HvCoorn_bVoltModRdyDrvRdyEna_C  SampleTime=-1
      settings: AttributesFormatString=%<Description>
  Calibration4 : Constant  Description=[0]  Value=HvCoorn_bVoltModHv2DftEna_C  SampleTime=-1
      settings: AttributesFormatString=%<Description>
  Calibration5 : Constant  Description=[0.3]  Value=HvCoorn_tiVoltModHv2DftReqThd_C  SampleTime=-1
      settings: AttributesFormatString=%<Description>
  Calibration6 : Constant  Description=[0]  Value=HvCoorn_bEmgyShtDwnReqEna_C  SampleTime=-1
      settings: AttributesFormatString=%<Description>
  ChgFull : Constant  Value=48  OutDataTypeStr=uint8
  Copyright : simulink/Model-Wide Utilities/Model Info  Frame=on  DisplayStringWithTags=|  HorizontalTextAlignment=Left  LeftAlignmentValue=0.02
      | © ITK Engineering Technology (Wu Xi) Co., Ltd. (ITKC)
      | 
      | Model Version: %<ModelVersion>
      | Date: %<LastModificationDate>
  Equal{1..2,4..10} (9 alike) : RelationalOperator  Operator===  OutDataTypeStr=boolean
  Equal3 : RelationalOperator  Operator=~=  OutDataTypeStr=boolean
  FALSE : Constant  Description=FALSE  Value=0  OutDataTypeStr=boolean
      settings: AttributesFormatString=%<Description>
  FALSE1 : Constant  Description=FALSE  Value=0  OutDataTypeStr=boolean
      settings: AttributesFormatString=%<Description>
  InlineDescription : ITKLib/Special/InlineDescription  Tag=HideFromReport  Description=电池模式请求  ShowInLibBrowser=0  RefreshPar=0
      settings: SourceProductName=ITKC_Lib
  Logical Operator1 : Logic  Inputs=5  AllPortsSameDT=off  OutDataTypeStr=boolean
  Logical Operator{6..10} (5 alike) : Logic  Operator=NOT  Inputs=1  AllPortsSameDT=off  OutDataTypeStr=boolean
  Logical Operator{2..3,11,14..15} (5 alike) : Logic  AllPortsSameDT=off  OutDataTypeStr=boolean
  Logical Operator12 : Logic  Operator=OR  AllPortsSameDT=off  OutDataTypeStr=boolean
  Logical Operator13 : Logic  Operator=OR  AllPortsSameDT=off  OutDataTypeStr=boolean
  Logical Operator4 : Logic  Inputs=6  AllPortsSameDT=off  OutDataTypeStr=boolean
  Logical Operator5 : Logic  Inputs=3  AllPortsSameDT=off  OutDataTypeStr=boolean
  OR{,1,3..6} (6 alike) : Logic  Operator=OR  OutDataTypeStr=boolean
  OR2 : Logic  Operator=OR  Inputs=3  OutDataTypeStr=boolean
  RSLatch : ITKLib/Memory/RSLatch
      settings: SourceProductName=ITKC_Lib
  Relational Operator1 : RelationalOperator  Operator===  OutDataTypeStr=boolean  InputSameDT=off
  Relational Operator2 : RelationalOperator  Operator=<  OutDataTypeStr=boolean  InputSameDT=off
  Relational Operator3 : RelationalOperator  OutDataTypeStr=boolean  InputSameDT=off
  Relational Operator4 : RelationalOperator  Operator=~=  OutDataTypeStr=boolean  InputSameDT=off
  Relational Operator5 : RelationalOperator  Operator=<  OutDataTypeStr=boolean  InputSameDT=off
  Relational Operator6 : RelationalOperator  OutDataTypeStr=boolean  InputSameDT=off
  Relational Operator7 : RelationalOperator  Operator=<  OutDataTypeStr=boolean  InputSameDT=off
  Relational Operator8 : RelationalOperator  Operator===  OutDataTypeStr=boolean  InputSameDT=off
  Relational Operator9 : RelationalOperator  Operator===  OutDataTypeStr=boolean  InputSameDT=off
  Switch{1..7} (7 alike) : Switch  Criteria=u2 ~= 0  SaturateOnIntegerOverflow=off  InputSameDT=off
  TRUE : Constant  Description=TRUE  OutDataTypeStr=boolean
      settings: AttributesFormatString=%<Description>
  TaskTime_s1 : Constant  Value=TaskTime_10ms
      settings: AttributesFormatString=[0.01]
  Turn_Off_Delay_Vari : ITKLib/TimeCounter/Turn_Off_Delay_Vari
      settings: AttributesFormatString=TurnOffDelay  SourceProductName=ITKC_Lib
  Unit Delay1 : UnitDelay  SampleTime=-1  HasFrameUpgradeWarning=on
      settings: AttributesFormatString=<initial=%<X0>>
  Unit Delay2 : UnitDelay  SampleTime=-1  HasFrameUpgradeWarning=on
      settings: AttributesFormatString=<initial=%<X0>>
  Unit detailed design : simulink/Model-Wide Utilities/DocBlock  Tag=HideFromReport  DocumentType=Text
      content=|
      | SMiVCU-3353 - 高压上电请求
      | 若<高压系统状态>大于等于12且小于101，则激活<高压上电请求>，否则若<高压系统状态>等于151，则<高压上电请求>保持上一时刻值，否则<高压上电请求>为0；
      |
      | SMiVCU-3358 - BMS模式请求
      | 满足以下全部条件，则<BMS模式请求>为0x4：DC charge：
      | 1.上一时刻<BMS模式请求>不为0x3：AC charge；
      | 2.<DC充电完成标志位>不为1；
      | 3.<高压上电请求>为1；
      | 4.<高压系统状态>小于90；
      | 5.<VCU内部充电状态>小于48；
      | 否则，满足以下全部条件，则<BMS模式请求>为0x3：AC charge：
      | 1.<AC充电完成标志位>不为1；
      | 2.<高压上电请求>为1；
      | 3.<高压系统状态>小于90；
      | 4.<VCU内部充电状态>小于48；
      | 5.<AC充电连接OK标志位>为1，则激活并锁存，待<AC充电连接标志位>为0则Reset。
      | 否则<高压上电请求>为1，<BMS模式请求>为0x2：Online；否则若<高压上电请求>为0，且<高压系统状态>大于151，则<BMS模式请求>为0x5:emergencyOffline；否则<BMS模式请求>为0x1：Offline。
      |
      | SMiVCU-3356 - 热管理使能标志位
      | <高压系统状态>等于89或90，则<热管理使能标志位>为1，否则为0。
      |
      | SMiVCU-3362 - 高压Ready标志位
      | <高压系统状态>等于90，则<高压Ready标志位>为1，否则为0。
      |
      | SMiVCU-3360 - DrvReady标志位
      | 若<VCU内部实际挡位状态>为0x5：R或0x4：D，且<高压系统状态>等于90，则<DrvReady标志位>为1，否则为0。
  UnitDelay : UnitDelay  SampleTime=-1  HasFrameUpgradeWarning=on
      settings: AttributesFormatString=<Initial=%<x0>>
  ocb_acCharge : Constant  Description=[3]  Value=BMSReqSt_ACChrg  OutDataTypeStr=uint8
      settings: AttributesFormatString=[3]
  ocb_acCharge1 : Constant  Description=[4]  Value=BMSReqSt_DCChrg  OutDataTypeStr=uint8
      settings: AttributesFormatString=[4]
  ocb_acCharge2 : Constant  Description=[3]  Value=BMSReqSt_ACChrg  OutDataTypeStr=uint8
      settings: AttributesFormatString=[3]
  ocb_emergencyOffline : Constant  Description=[5]  Value=BMSReqSt_emergencyOffline  OutDataTypeStr=uint8
      settings: AttributesFormatString=[5]
  ocb_offline : Constant  Description=[1]  Value=BMSReqSt_offline  OutDataTypeStr=uint8
      settings: AttributesFormatString=[1]
  ocb_online : Constant  Description=[2]  Value=BMSReqSt_online  OutDataTypeStr=uint8
      settings: AttributesFormatString=[2]
  ocm_discharge1 : Constant  Description=[4]  Value=VoltMod_stHvReq_SC  OutDataTypeStr=uint8
      settings: AttributesFormatString=%<Description>
  ocm_discharge10 : Constant  Description=[0]  Value=VoltMod_stDft_SC  OutDataTypeStr=uint8
      settings: AttributesFormatString=%<Description>
  ocm_discharge2 : Constant  Description=[3]  Value=VoltMod_stHvDcnct_SC  OutDataTypeStr=uint8
      settings: AttributesFormatString=%<Description>
  ocm_discharge3 : Constant  Description=[5]  Value=GearLvr_stDrvGearR_SC  OutDataTypeStr=uint8
      settings: AttributesFormatString=%<Description>
  ocm_discharge4 : Constant  Description=[5]  Value=VoltMod_stVoltModRdy_SC  OutDataTypeStr=uint8
      settings: AttributesFormatString=%<Description>
  ocm_discharge5 : Constant  Description=[1]  Value=GearLvr_stDrvGearD_SC  OutDataTypeStr=uint8
      settings: AttributesFormatString=%<Description>
  ocm_discharge6 : Constant  Description=[5]  Value=VoltMod_stVoltModRdy_SC  OutDataTypeStr=uint8
      settings: AttributesFormatString=%<Description>
  ocm_discharge7 : Constant  Description=[8]  Value=VoltMod_stDCBuck_SC  OutDataTypeStr=uint8
      settings: AttributesFormatString=%<Description>
  ocm_discharge8 : Constant  Description=[7]  Value=VoltMod_stHvCnt_SC  OutDataTypeStr=uint8
      settings: AttributesFormatString=%<Description>
  ocm_discharge9 : Constant  Description=[5]  Value=VoltMod_stVoltModRdy_SC  OutDataTypeStr=uint8
      settings: AttributesFormatString=%<Description>
  uint1 : Constant  Description=Shutdown_HV  Value=101  OutDataTypeStr=uint8
      settings: AttributesFormatString=|
      | %<OutDataTypeStr>
      | %<Description>
  uint2 : Constant  Description=SystemEmergencyShutDown  Value=151  OutDataTypeStr=uint8
      settings: AttributesFormatString=|
      | %<OutDataTypeStr>
      | %<Description>
  uint3 : Constant  Description=Ready  Value=90  OutDataTypeStr=uint8
      settings: AttributesFormatString=|
      | %<OutDataTypeStr>
      | %<Description>
  uint4 : Constant  Description=SystemEmergencyShutDown  Value=151  OutDataTypeStr=uint8
      settings: AttributesFormatString=|
      | %<OutDataTypeStr>
      | %<Description>
  uint5 : Constant  Description=Ready  Value=90  OutDataTypeStr=uint8
      settings: AttributesFormatString=|
      | %<OutDataTypeStr>
      | %<Description>
  uint6 : Constant  Description=ReadyWait  Value=89  OutDataTypeStr=uint8
      settings: AttributesFormatString=|
      | %<OutDataTypeStr>
      | %<Description>
  uint8 : Constant  Description=HvContactorRequest  Value=12  OutDataTypeStr=uint8
      settings: AttributesFormatString=|
      | %<OutDataTypeStr>
      | %<Description>
  HvCoorn_bHvOnReq : Outport  VectorParamsAs1DForOutWhenUnconnected=off
  HvCoorn_stBMSModeReq : Outport  Port=2  VectorParamsAs1DForOutWhenUnconnected=off
  HvCoorn_bHvReady : Outport  Port=3  VectorParamsAs1DForOutWhenUnconnected=off
  HvCoorn_bDrvRdy : Outport  Port=4
  HvCoorn_bEccEna : Outport  Port=5  VectorParamsAs1DForOutWhenUnconnected=off
  HvCoorn_bRdyLamp : Outport  Port=6
  wires:
  uint8/1 -> Relational Operator3/2
  HvCoorn_stHVP/1 -> Relational Operator3/1, Relational Operator8/1, Relational Operator9/1, Relational Operator6/1, Relational Operator5/1, Relational Operator1/1, Relational Operator2/1
  uint1/1 -> Relational Operator2/2
  Relational Operator3/1 -> Logical Operator2/1
  Relational Operator2/1 -> Logical Operator2/2
  uint2/1 -> Relational Operator1/2
  TRUE/1 -> Switch3/1
  Unit Delay2/1 -> Switch1/1
  FALSE/1 -> Switch1/3
  Switch1/1 -> Switch3/3
  Switch4/1 -> Unit Delay1/1, HvCoorn_stBMSModeReq/1
  ocb_acCharge/1 -> Switch2/1
  Switch5/1 -> Switch2/3
  ocb_online/1 -> Switch5/1
  Switch6/1 -> Switch5/3
  ocb_emergencyOffline/1 -> Switch6/1
  Logical Operator7/1 -> Logical Operator3/1
  Relational Operator6/1 -> Logical Operator3/2
  Logical Operator3/1 -> Switch6/2
  ocb_offline/1 -> Switch6/3
  Logical Operator1/1 -> Switch2/2
  uint3/1 -> Relational Operator5/2
  Relational Operator5/1 -> [NotReady]
  Chrg_stChrg/1 -> Relational Operator7/1
  ChgFull/1 -> Relational Operator7/2
  Relational Operator7/1 -> Logical Operator4/6, Logical Operator1/1
  HvCoorn_bACChrgLink/1 -> Logical Operator6/1
  Logical Operator6/1 -> RSLatch/2
  HvCoorn_bACChrgLinkOk/1 -> RSLatch/1
  RSLatch/1 -> Logical Operator1/5
  Chrg_bACChrgCmpl/1 -> Logical Operator8/1
  Logical Operator8/1 -> Logical Operator1/4
  uint4/1 -> Relational Operator6/2
  Chrg_bDCChrgCmpl/1 -> Logical Operator9/1
  icbms_bDcChrgCfg/1 -> Logical Operator4/2
  Switch2/1 -> Switch4/3
  Logical Operator4/1 -> Switch4/2
  ocb_acCharge1/1 -> Switch4/1
  ocb_acCharge2/1 -> Relational Operator4/2
  Unit Delay1/1 -> Relational Operator4/1
  Relational Operator4/1 -> Logical Operator4/1
  Logical Operator9/1 -> Logical Operator4/3
  [NotReady] -> Logical Operator1/2
  [NotReady] -> Logical Operator4/5
  uint5/1 -> Relational Operator8/2
  ocm_discharge3/1 -> Equal4/2
  ocm_discharge5/1 -> Equal6/2
  OR/1 -> AND1/3
  GearLvr_stDrvGear/1 -> Equal6/1, Equal4/1
  Equal4/1 -> OR/1
  Equal6/1 -> OR/2
  Relational Operator8/1 -> OR5/1, OR1/2
  Relational Operator9/1 -> OR1/1
  uint6/1 -> Relational Operator9/2
  OR1/1 -> HvCoorn_bHvReady/1, Logical Operator5/2
  Logical Operator5/1 -> HvCoorn_bEccEna/1
  HvCoorn_bVoltModStbReq/1 -> Logical Operator10/1
  Logical Operator10/1 -> AND1/1, Logical Operator13/1, Logical Operator5/3
  Switch7/1 -> Switch5/2, Logical Operator7/1, Logical Operator1/3, Logical Operator4/4, Unit Delay2/1, HvCoorn_bHvOnReq/1
  Equal2/1 -> OR2/2
  Equal1/1 -> OR2/1
  ocm_discharge1/1 -> Equal1/2
  ocm_discharge2/1 -> Equal2/2
  [HvCoorn_stVoltMod] -> Equal3/1
  ocm_discharge4/1 -> Equal3/2
  Equal3/1 -> Logical Operator12/1
  Logical Operator12/1 -> Logical Operator5/1
  Calibration1/1 -> Logical Operator12/2
  AND1/1 -> HvCoorn_bRdyLamp/1
  Switch3/1 -> Switch7/3
  FALSE1/1 -> Switch7/1
  Equal5/1 -> OR2/3
  ocm_discharge6/1 -> Equal5/2
  Logical Operator2/1 -> OR3/2
  OR3/1 -> Switch3/2
  OR4/1 -> OR3/1
  ocm_discharge7/1 -> Equal7/2
  Equal7/1 -> OR4/2
  ocm_discharge8/1 -> Equal8/2
  HvCoorn_stVoltMod/1 -> [HvCoorn_stVoltMod], Equal1/1, Equal2/1, Equal5/1, Equal7/1, Equal8/1, Equal10/1
  Equal8/1 -> OR4/1
  Logical Operator11/1 -> HvCoorn_bDrvRdy/1
  Calibration2/1 -> Logical Operator13/2
  Logical Operator13/1 -> Logical Operator11/2
  ocm_discharge9/1 -> Equal9/2
  [HvCoorn_stVoltMod] -> Equal9/1
  Equal9/1 -> Logical Operator14/1
  Calibration3/1 -> Logical Operator14/2
  Logical Operator14/1 -> OR5/2
  OR5/1 -> AND1/2, Logical Operator11/1
  OR2/1 -> OR6/1, UnitDelay/1
  OR6/1 -> Switch7/2
  UnitDelay/1 -> AND/1
  ocm_discharge10/1 -> Equal10/2
  Equal10/1 -> AND/2
  Calibration4/1 -> AND/3
  Turn_Off_Delay_Vari/1 -> OR6/2
  AND/1 -> Turn_Off_Delay_Vari/1
  TaskTime_s1/1 -> Turn_Off_Delay_Vari/2
  Calibration5/1 -> Turn_Off_Delay_Vari/3
  Relational Operator1/1 -> Logical Operator15/1
  Logical Operator15/1 -> Switch1/2
  Calibration6/1 -> Logical Operator15/2
